simulink model "untitled"  (R2021b)
settings: Solver=VariableStepAuto  StartTime=0.0  StopTime=10.0  MaxStep=0.02  MinStep=0.01  RelTol=1e-3
undefined symbols (not defined in the file or in its folder): anal_den, anal_num, g, maxRotorLift, weight, wn, zeta
settings Model: Creator=chris  LastModifiedBy=chris

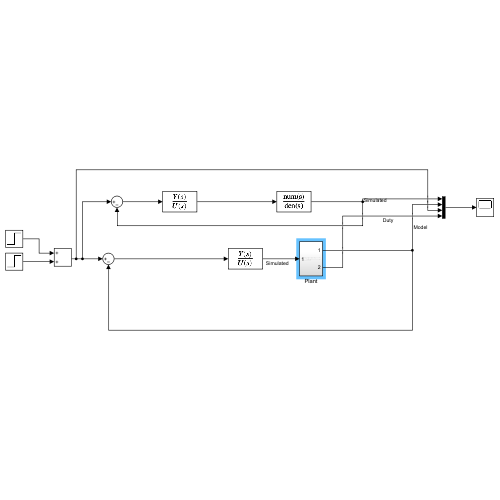
[thumbnail: Simulink's stored preview of the top-level diagram]
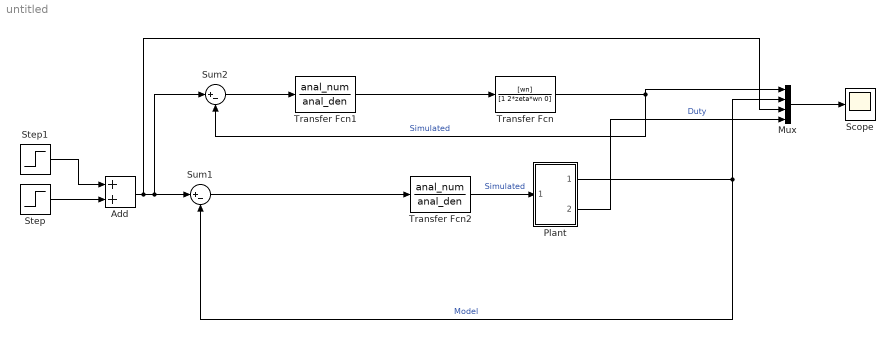
== system untitled ==
  Add : Sum
  Mux : Mux
  Plant : Subsystem
  Scope : Scope
  Step : Step  SampleTime=0
  Step1 : Step  Time=0  After=0  SampleTime=0
  Sum1 : Sum  Inputs=|+-
  Sum2 : Sum  Inputs=|+-
  Transfer Fcn : TransferFcn  Numerator=[wn]  Denominator=[1 2*zeta*wn 0]
  Transfer Fcn1 : TransferFcn  Numerator=anal_num  Denominator=anal_den
  Transfer Fcn2 : TransferFcn  Numerator=anal_num  Denominator=anal_den
  wires:
  Step/1 -> Add/2
  Add/1 -> Mux/3, Sum2/1, Sum1/1
  Step1/1 -> Add/1
  Plant/1(Out1) -> Sum1/2, Mux/2  "Model"
  Sum1/1 -> Transfer Fcn2/1
  Sum2/1 -> Transfer Fcn1/1
  Transfer Fcn/1 -> Sum2/2, Mux/1  "Simulated"
  Mux/1 -> Scope/1
  Transfer Fcn1/1 -> Transfer Fcn/1
  Plant/2(Out2) -> Mux/4  "Duty"
  Transfer Fcn2/1 -> Plant/1(In1)  "Simulated"

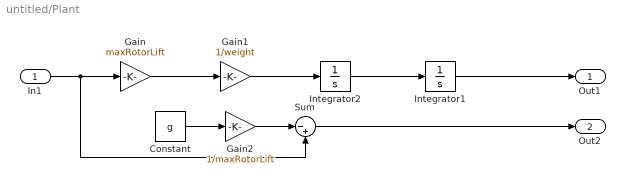
== system untitled/Plant ==
  In1 : Inport
  Constant : Constant  Value=g
  Gain : Gain  Gain=maxRotorLift
  Gain1 : Gain  Gain=1/weight
  Gain2 : Gain  Gain=1/maxRotorLift
  Integrator1 : Integrator
  Integrator2 : Integrator
  Sum : Sum  Inputs=|-+
  Out1 : Outport
  Out2 : Outport  Port=2
  wires:
  Gain/1 -> Gain1/1
  Integrator2/1 -> Integrator1/1
  Integrator1/1 -> Out1/1
  In1/1 -> Sum/2, Gain/1
  Constant/1 -> Gain2/1
  Gain1/1 -> Integrator2/1
  Gain2/1 -> Sum/1
  Sum/1 -> Out2/1
